simulink model "simulink_model"  (R2013b)
settings: Solver=ode45  StartTime=0.0  StopTime=30  RelTol=1e-3
settings Model: Creator=petter  LastModifiedBy=petter

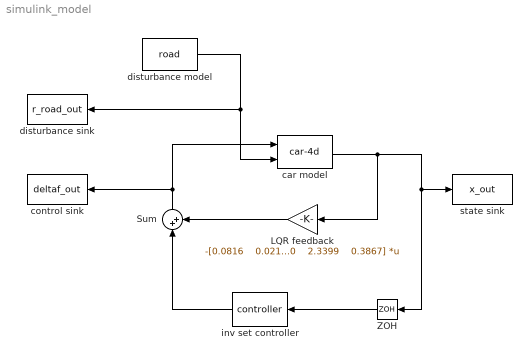
== system simulink_model ==
  LQR feedback : Gain  Gain="-[0.0816    0.0210    2.3399    0.3867]"  Multiplication=Matrix(K*u)  SampleTime=0
  Sum : Sum  Inputs=|++  SampleTime=0
  ZOH : ZeroOrderHold  SampleTime=0.05
  car model : M-S-Function  FunctionName=car-4d
  control sink : ToWorkspace  VariableName=deltaf_out  SampleTime=-1  SaveFormat=Structure With Time
  disturbance model : M-S-Function  FunctionName=road
  disturbance sink : ToWorkspace  VariableName=r_road_out  SampleTime=-1  SaveFormat=Structure With Time
  inv set controller : M-S-Function  FunctionName=controller  Parameters=1
  state sink : ToWorkspace  VariableName=x_out  SampleTime=-1  SaveFormat=Structure With Time
  wires:
  car model/1 -> LQR feedback/1, ZOH/1, state sink/1
  inv set controller/1 -> Sum/1
  disturbance model/1 -> disturbance sink/1, car model/2
  ZOH/1 -> inv set controller/1
  LQR feedback/1 -> Sum/2
  Sum/1 -> control sink/1, car model/1
